simulink model "StSys_StrtRmp"  (R2016b)
settings: configuration reference "CodeGenConfigSet" (kept outside this file)
values from neighbouring files (symbols this model uses):
  StSys_trqStrtMax_CUR = Calibration.Parameter    [init_StSys_StrtRmp.m]
  StSys_trqStrtMax_CURX = Calibration.Parameter    [init_StSys_StrtRmp.m]
  TRQ_ZERO = fi(0,Trq_Nm)    [init_StSys_StrtRmp.m]
settings Model: Creator=Colin  LastModifiedBy=lenovo
settings ConfigSetRef: SourceLocation=Base Workspace

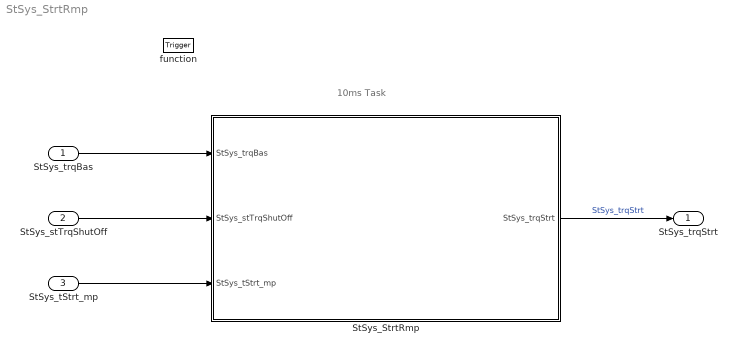
== system StSys_StrtRmp ==
  note: 10ms Task
  StSys_trqBas : Inport  Tag=Nm  Description=basic starting torque  OutMin=0  OutMax=1000  OutDataTypeStr=Trq_Nm
  StSys_stTrqShutOff : Inport  Tag=[]  Description=the status of the starting torque shuto-off input  Port=2  OutMin=0  OutMax=1  OutDataTypeStr=boolean
  StSys_tStrt_mp : Inport  Tag=deg  Description=engine temperature for starting system  Port=3  OutMin=-50  OutMax=150  OutDataTypeStr=Temp_deg
  function : TriggerPort  TriggerType=function-call  VariantControl=Variant
  StSys_StrtRmp : Subsystem
  StSys_trqStrt : Outport  Tag=Nm  Description=Engine starting torque  OutMin=-3000  OutMax=3000  OutDataTypeStr=Trq_Nm
  wires:
  StSys_trqBas/1 -> StSys_StrtRmp/1(StSys_trqBas)
  StSys_tStrt_mp/1 -> StSys_StrtRmp/3(StSys_tStrt_mp)
  StSys_stTrqShutOff/1 -> StSys_StrtRmp/2(StSys_stTrqShutOff)
  StSys_StrtRmp/1(StSys_trqStrt) -> StSys_trqStrt/1  "StSys_trqStrt"

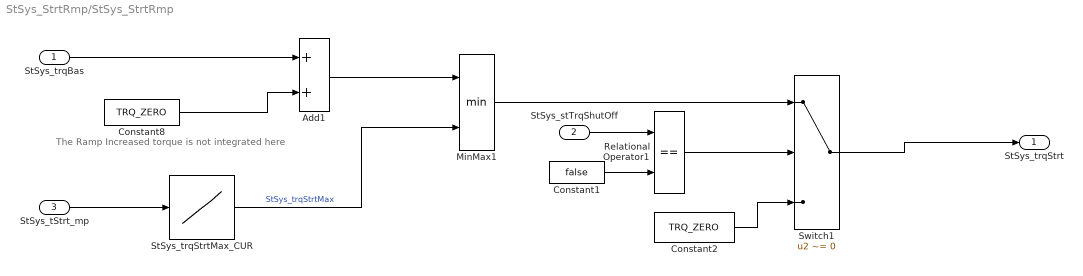
== system StSys_StrtRmp/StSys_StrtRmp ==
  note: The Ramp Increased torque is not integrated here
  StSys_trqBas : Inport
  StSys_stTrqShutOff : Inport  Port=2
  StSys_tStrt_mp : Inport  Tag=deg  Description=engine temperature for starting system  Port=3  OutMin=-50  OutMax=150  OutDataTypeStr=Temp_deg
  Add1 : Sum
  Constant1 : Constant  Value=false
  Constant2 : Constant  Value=TRQ_ZERO  OutDataTypeStr=Trq_Nm
  Constant8 : Constant  Value=TRQ_ZERO  OutDataTypeStr=Trq_Nm
  MinMax1 : MinMax  Inputs=2  InputSameDT=on
  Relational Operator1 : RelationalOperator  Operator===  OutDataTypeStr=boolean  RndMeth=Simplest
  StSys_trqStrtMax_CUR : Lookup_n-D  NumberOfTableDimensions=1  BreakpointsForDimension1=StSys_trqStrtMax_CURX  BreakpointsForDimension1DataTypeStr=Temp_deg  IndexSearchMethod=Linear search  Table=StSys_trqStrtMax_CUR  TableDataTypeStr=Trq_Nm  ExtrapMethod=Clip  InternalRulePriority=Speed  OutDataTypeStr=Trq_Nm  RndMeth=Simplest  InputSameDT=on
  Switch1 : Switch  Criteria=u2 ~= 0
  StSys_trqStrt : Outport  PortDimensions=1
  wires:
  Switch1/1 -> StSys_trqStrt/1
  StSys_tStrt_mp/1 -> StSys_trqStrtMax_CUR/1
  Constant8/1 -> Add1/2
  StSys_trqBas/1 -> Add1/1
  Add1/1 -> MinMax1/1
  StSys_trqStrtMax_CUR/1 -> MinMax1/2  "StSys_trqStrtMax"
  MinMax1/1 -> Switch1/1
  Constant2/1 -> Switch1/3
  Relational Operator1/1 -> Switch1/2
  Constant1/1 -> Relational Operator1/2
  StSys_stTrqShutOff/1 -> Relational Operator1/1
